simulink model "fallschirm3"  (R2019b)
settings: Solver=ode45  StartTime=0.0  StopTime=inf  RelTol=1e-3  EnableMultiTasking=on
model workspace (MAT data in the model file):
  AFS = 30
  AS = 0.5
  cw = 1.3
  g = 9.81
  h0 = 500
  h1 = 100
  m = 85
  rho = 1.2
  v0 = 0
settings Model: Creator=Reichl  LastModifiedBy=jakob
settings DataIOCC: SaveFormat=Array  ReturnWorkspaceOutputs=off
settings OptimizationCC: LifeSpan=inf
settings DebuggingCC: AllowSymbolicDim=off  SFUnexpectedBacktrackingDiag=warning  SFNoUnconditionalDefaultTransitionDiag=warning  SFExecutionAtInitializationDiag=none  ArithmeticOperatorsInVariantConditions=warning
settings HardwareCC: ProdBitPerPointer=32  ProdBitPerSizeT=32  ProdBitPerPtrDiffT=32  ProdLargestAtomicFloat=None  ProdIntDivRoundTo=Undefined  ProdEndianess=Unspecified  ProdWordSize=32  ProdHWDeviceType=32-bit Generic
settings ModelReferenceCC: PropagateSignalLabelsOutOfModel=off
settings SFSimCC: SimUseLocalCustomCode=off  CustomCodeUndefinedFunction=UseInterfaceOnly
settings RTWCC: RTWUseLocalCustomCode=off
settings CodeAppCC: StateflowObjectComments=on
settings GRTTargetCC: TargetLangStandard=C89/C90 (ANSI)  GeneratePreprocessorConditionals=Disable all
settings ConfigComp: CovMetricSettings=dw  CovHtmlReporting=on  CovSaveCumulativeToWorkspaceVar=on  CovSaveSingleToWorkspaceVar=on  CovExternalEMLEnable=off  CovSFcnEnable=off

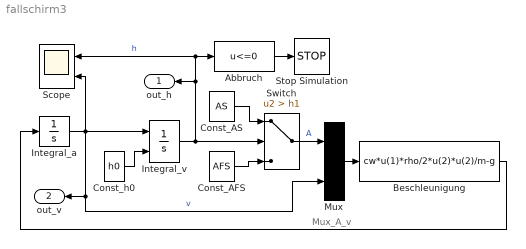
== system fallschirm3 ==
  note: Mux_A_v
  Abbruch : Fcn  Expr=u<=0
  Beschleunigung : Fcn  Expr=cw*u(1)*rho/2*u(2)*u(2)/m-g
  Const_AFS : Constant  Value=AFS
  Const_AS : Constant  Value=AS
  Const_h0 : Constant  Value=h0
  Integral_a : Integrator  InitialCondition=v0
  Integral_v : Integrator  InitialConditionSource=external
  Mux : Mux  Inputs=2
      settings: DisplayOption=signals
  Scope : Scope  NumInputPorts=2
  Stop Simulation : Stop
  Switch : Switch  Criteria=u2 > Threshold  Threshold=h1  ZeroCross=off
  out_h : Outport  VectorParamsAs1DForOutWhenUnconnected=off
  out_v : Outport  Port=2  VectorParamsAs1DForOutWhenUnconnected=off
  wires:
  Integral_a/1 -> Scope/2, Integral_v/1, out_v/1, Mux/2  "v"
  Integral_v/1 -> Switch/2, out_h/1, Scope/1, Abbruch/1  "h"
  Const_AS/1 -> Switch/1
  Const_AFS/1 -> Switch/3
  Switch/1 -> Mux/1  "A"
  Abbruch/1 -> Stop Simulation/1
  Const_h0/1 -> Integral_v/2
  Mux/1 -> Beschleunigung/1
  Beschleunigung/1 -> Integral_a/1
